simulink model "wind_turbine_design_and_simulation"  (R2019b)
settings: Solver=ode23tb  StartTime=0.0  StopTime=60.0  FixedStep=0.001  MaxStep=1/60  RelTol=1e-3  AbsTol=1e-3
libraries: powerlib x9, powerlib_meascontrol x2, re_lib x1
settings Model: Creator=USER  LastModifiedBy=USER
settings SolverCC: AutoScaleAbsTol=off  SolverResetMethod=Robust

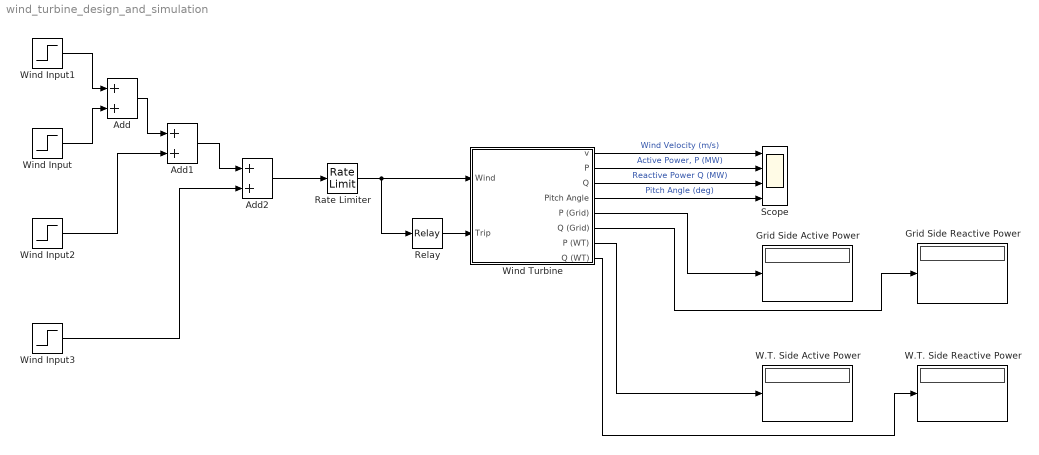
== system wind_turbine_design_and_simulation ==
  Add : Sum
  Add1 : Sum
  Add2 : Sum
  Grid Side Active Power : Display
  Grid Side Reactive Power : Display
  Rate Limiter : RateLimiter
  Relay : Relay  OnSwitchValue=15  OffSwitchValue=0
      settings: AttributesFormatString=On at %<OnSwitchValue>m/s
  Scope : Scope  NumInputPorts=4
  W.T. Side Active Power : Display
  W.T. Side Reactive Power : Display
  Wind Input : Step  Time=20  SampleTime=0
      settings: AttributesFormatString=|
      | %<Before>m/s to %<After>m/s
      | at %<Time>s
  Wind Input1 : Step  Time=10  Before=6  After=8  SampleTime=0
      settings: AttributesFormatString=|
      | %<Before>m/s to %<After>m/s
      | at %<Time>s
  Wind Input2 : Step  Time=30  After=3  SampleTime=0
      settings: AttributesFormatString=|
      | %<Before>m/s to %<After>m/s
      | at %<Time>s
  Wind Input3 : Step  Time=45  After=3  SampleTime=0
      settings: AttributesFormatString=|
      | %<Before>m/s to %<After>m/s
      | at %<Time>s
  Wind Turbine : Subsystem
  wires:
  Wind Turbine/2(P) -> Scope/2  "Active Power, P (MW)"
  Wind Turbine/3(Q) -> Scope/3  "Reactive Power Q (MW)"
  Wind Turbine/4(Pitch Angle) -> Scope/4  "Pitch Angle (deg)"
  Wind Turbine/1(v) -> Scope/1  "Wind Velocity (m/s)"
  Wind Turbine/5(P (Grid)) -> Grid Side Active Power/1
  Wind Turbine/6(Q (Grid)) -> Grid Side Reactive Power/1
  Wind Turbine/7(P (WT)) -> W.T. Side Active Power/1
  Wind Turbine/8(Q (WT)) -> W.T. Side Reactive Power/1
  Relay/1 -> Wind Turbine/2(Trip)
  Wind Input/1 -> Add/2
  Wind Input3/1 -> Add2/2
  Wind Input1/1 -> Add/1
  Add/1 -> Add1/1
  Add2/1 -> Rate Limiter/1
  Wind Input2/1 -> Add1/2
  Rate Limiter/1 -> Wind Turbine/1(Wind), Relay/1
  Add1/1 -> Add2/1

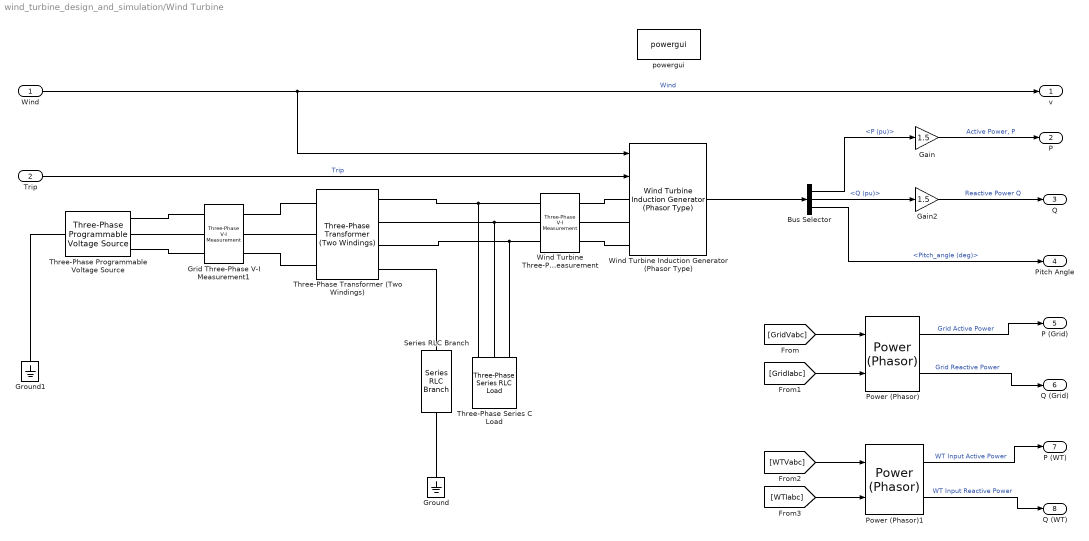
== system wind_turbine_design_and_simulation/Wind Turbine ==
  Wind : Inport
  Trip : Inport  Port=2
  Bus Selector : BusSelector  OutputSignals=P (pu),Q (pu),Pitch_angle (deg)
  Gain : Gain  Gain=1.5
  Gain2 : Gain  Gain=1.5
  Grid Three-Phase V-I Measurement1 : powerlib/Measurements/Three-Phase V-I Measurement  VoltageMeasurement=phase-to-ground  SetLabelV=on  LabelV=GridVabc  Vpu=off  VpuLL=off  CurrentMeasurement=yes  SetLabelI=on  LabelI=GridIabc  Ipu=off  Pbase=100e6  Vbase=500e3  OutputType=Complex  PhasorSimulation=on  PSBequivalent=0
      settings: SourceProductName=Simscape Electrical
  Ground : powerlib/Elements/Ground  LConnTagsString=a
      settings: SourceProductName=Simscape Electrical
  Ground1 : powerlib/Elements/Ground  LConnTagsString=a
      settings: SourceProductName=Simscape Electrical
  Power (Phasor) : powerlib_meascontrol/Measurements/Power (Phasor)
      settings: SourceProductName=Simscape Electrical  SourceProductBaseCode=PS
  Power (Phasor)1 : powerlib_meascontrol/Measurements/Power (Phasor)
      settings: SourceProductName=Simscape Electrical  SourceProductBaseCode=PS
  Series RLC Branch : powerlib/Elements/Series RLC Branch  LConnTagsString=__new0  RConnTagsString=__new0  BranchType=R  Resistance=66  Inductance=1e-3  SetiL0=off  InitialCurrent=0  Capacitance=1e-6  Setx0=off  InitialVoltage=0  Measurements=None
      settings: AttributesFormatString=%<Resistance> Ohms  SourceProductName=Simscape Electrical
  Three-Phase Programmable Voltage Source : powerlib/Electrical Sources/Three-Phase Programmable Voltage Source  PositiveSequence="[25e3  0 60]"  VariationEntity=None  VariationType=Table of time-amplitude pairs  VariationTypeAlt=Step  VariationStep=0.5  VariationRate=10  VariationMagnitude=0.3  VariationFrequency=2  VariationTiming=[1 2]  VariationPhaseA=off  Amplitudes=[1 0.8 1.2 1.0]  TimeValues=[0 0.1 0.15 0.2]  HarmonicGeneration=off  HarmonicA=[3 0.2 -25 0]  HarmonicB=[2 0.15 35 2]  Timing="[0.05  3]"  BusType=swing  Pref=0  Qref=0  Qmin=-inf  Qmax=inf
      settings: AttributesFormatString=%<PositiveSequence>  SourceProductName=Simscape Electrical
  Three-Phase Series C Load : powerlib/Elements/Three-Phase Series RLC Load  LConnTagsString=A|B|C  Configuration=Delta  NominalVoltage=575  Vabc=[1e3 1e3 1e3]  Vabcp=[1e3 1e3 1e3]  NominalFrequency=60  UnbalancedPower=off  ActivePower=0  InductivePower=0  CapacitivePower=400e3  Pabc=[10e3 9e3 11e3]  QLabc=[100 90 110]  QCabc=[100 90 110]  Pabcp=[10e3 9e3 11e3]  QLabcp=[100 90 110]  QCabcp=[100 90 110]  Measurements=None  LoadType=constant Z
      settings: AttributesFormatString=%<CapacitivePower>Qc  SourceProductName=Simscape Electrical
  Three-Phase Transformer (Two Windings) : powerlib/Elements/Three-Phase Transformer (Two Windings)  Winding1Connection=Yg  Winding2Connection=Yn  CoreType=Three single-phase transformers  SetSaturation=off  Hysteresis=off  DataFile='hysteresis'  SetInitialFlux=off  Measurements=None  UNITS=pu  NominalPower=[ 4e6 , 60 ]  Winding1=[ 25e3 , 0.025/10 , 0.025 ]  Winding2=[ 575 , 0.025/30 , 0.025 ]  Rm=500  Lm=inf  L0=0.49999  Saturation=[ 0,0 ; 0.0024,1.2 ; 1.0,1.52 ]  InitialFluxes=[0.79999 -0.79999 0.7]  BreakLoop=off  DiscreteSolver=Trapezoidal iterative  DataType=off  TransfoNumber=1
      settings: SourceProductName=Simscape Electrical
      settings: AttributesFormatString=|
      | In: %<Winding1>
      | Out: %<Winding2>
      | Nominal P and freq: %<NominalPower>
  Wind Turbine Induction Generator (Phasor Type) : re_lib/Wind Generation/Wind Turbine Induction Generator (Phasor Type)  ExternalTm=off  nom=[1.5e6, 575, 60]  sta=[ 0.004843, 0.1248]  rot=[ 0.004377, 0.1791]  Lm=6.77  mec=[5.04, 0.01, 3]  init="[ -0.01,0,   0,0,0,   0,0,0 ]"  pitch_angle=0  Pmec=1.5e6  wind_base=9  speed_nom=1  P_wind_base=1  K_pitch_gain=[5 25]  pitch_max=45  pitch_rate=2
      settings: SourceProductName=Simscape Electrical  SourceProductBaseCode=PS
      settings: AttributesFormatString=|
      | Nominal Power: %<Pmec>W
      | Base Wind Speed: %<wind_base>m/s
  Wind Turbine Three-Phase V-I Measurement : powerlib/Measurements/Three-Phase V-I Measurement  VoltageMeasurement=phase-to-ground  SetLabelV=on  LabelV=WTVabc  Vpu=off  VpuLL=off  CurrentMeasurement=yes  SetLabelI=on  LabelI=WTIabc  Ipu=off  Pbase=100e6  Vbase=500e3  OutputType=Complex  PhasorSimulation=on  PSBequivalent=0
      settings: SourceProductName=Simscape Electrical
  powergui : powerlib/powergui  Priority=1  SimulationMode=Phasor  SampleTime=50e-6  frequency=60  Iterations=50  frequencyindice=60  Pbase=10e6  ErrMax=1e-4  UnitsV=V  UnitsW=W  buscounter=0  FunctionMessages=off  echomessages=off  EnableUseOfTLC=off  CurrentSourceSwitches=off  DisableSnubberDevices=off  DisableRonSwitches=off  DisableVfSwitches=off  DisplayEquations=off  AutomaticDiscreteSolvers=off  SolverType=Tustin/Backward Euler (TBE)  Interpol=off  ExternalGateDelay=off  methode=off  Ts=100  x0status=blocks  SPID=on  SwTol=0  HookPort=off  NonlinearTolerance=1e-4  nMaxIteration=100  ContinueOnMaxIteration=off  RestoreLinks=warning  ResistiveCurrentMeasurement=off  Frange=[0:2:500]  Ylog=off  Xlog=on  ShowGrid=off  save=off  variable=ZData  structure=0  ZoomFFT=off  StartTime=0.0  cycles=1  DisplayStyle=1  fundamental=60  FreqAxis=off  MaxFrequency=1000  frequencyindicesteady=1  RmsSteady=1  display=off
      settings: SourceProductName=Simscape Electrical
  v : Outport
  P : Outport  Port=2
  Q : Outport  Port=3
  Pitch Angle : Outport  Port=4
  P (Grid) : Outport  Port=5
  Q (Grid) : Outport  Port=6
  P (WT) : Outport  Port=7
  Q (WT) : Outport  Port=8
  wires:
  Wind Turbine Induction Generator (Phasor Type)/1 -> Bus Selector/1
  Trip/1 -> Wind Turbine Induction Generator (Phasor Type)/2  "Trip"
  Bus Selector/2 -> Gain2/1  "<Q (pu)>"
  Bus Selector/3 -> Pitch Angle/1  "<Pitch_angle (deg)>"
  Gain2/1 -> Q/1  "Reactive Power Q"
  Bus Selector/1 -> Gain/1  "<P (pu)>"
  Gain/1 -> P/1  "Active Power, P"
  Wind/1 -> Wind Turbine Induction Generator (Phasor Type)/1, v/1  "Wind"
  [GridVabc] -> Power (Phasor)/1
  [GridIabc] -> Power (Phasor)/2
  [WTVabc] -> Power (Phasor)1/1
  [WTIabc] -> Power (Phasor)1/2
  Power (Phasor)/1 -> P (Grid)/1  "Grid Active Power"
  Power (Phasor)/2 -> Q (Grid)/1  "Grid Reactive Power"
  Power (Phasor)1/1 -> P (WT)/1  "WT Input Active Power"
  Power (Phasor)1/2 -> Q (WT)/1  "WT Input Reactive Power"
  connections:
  Grid Three-Phase V-I Measurement1/RConn1 -- Three-Phase Transformer (Two Windings)/LConn1
  Series RLC Branch/RConn1 -- Ground/LConn1
  Three-Phase Transformer (Two Windings)/RConn4 -- Series RLC Branch/LConn1
  Grid Three-Phase V-I Measurement1/RConn2 -- Three-Phase Transformer (Two Windings)/LConn2
  Grid Three-Phase V-I Measurement1/RConn3 -- Three-Phase Transformer (Two Windings)/LConn3
  Three-Phase Programmable Voltage Source/LConn1 -- Ground1/LConn1
  Grid Three-Phase V-I Measurement1/LConn2 -- Three-Phase Programmable Voltage Source/RConn2
  Three-Phase Programmable Voltage Source/RConn1 -- Grid Three-Phase V-I Measurement1/LConn1
  Three-Phase Programmable Voltage Source/RConn3 -- Grid Three-Phase V-I Measurement1/LConn3
  Wind Turbine Three-Phase V-I Measurement/RConn1 -- Wind Turbine Induction Generator (Phasor Type)/LConn1
  Wind Turbine Three-Phase V-I Measurement/RConn2 -- Wind Turbine Induction Generator (Phasor Type)/LConn2
  Wind Turbine Three-Phase V-I Measurement/RConn3 -- Wind Turbine Induction Generator (Phasor Type)/LConn3
  Three-Phase Transformer (Two Windings)/RConn1 -- Three-Phase Series C Load/LConn1 -- Wind Turbine Three-Phase V-I Measurement/LConn1
  Three-Phase Transformer (Two Windings)/RConn2 -- Three-Phase Series C Load/LConn2 -- Wind Turbine Three-Phase V-I Measurement/LConn2
  Three-Phase Transformer (Two Windings)/RConn3 -- Three-Phase Series C Load/LConn3 -- Wind Turbine Three-Phase V-I Measurement/LConn3
